simulink model "Drone_BBall_Developer"  (R2020a)
settings: Solver=FixedStepAuto  StartTime=0.0  StopTime=60  FixedStep=.001  RelTol=1e-3
values from neighbouring files (symbols this model uses):
  b = .25*m    (= 0.25)    [Run_Match.m]
  b_ball = .02*m_ball    (= 0.01)    [Run_Match.m]
  b_F_hook = 100    [Run_Match.m]
  b_F_hoop = m_ball * 50    (= 25)    [Run_Match.m]
  b_F_R = m * 20    (= 20)    [Run_Match.m]
  b_F_R_ball = m_ball * 10    (= 5)    [Run_Match.m]
  b_F_R_hook = m_hook * 100    (= 10)    [Run_Match.m]
  B_hook = r_hook^2*6*m_ball*g    (= 0.2943)    [Run_Match.m]
  b_hook = 0.05*m_hook    (= 0.005)    [Run_Match.m]
  b_tether = 1    [Run_Match.m]
  b_th = .1*J    (= 0.0192708333333)    [Run_Match.m]
  b_th_ball = .05*J_ball    (= 0.0009)    [Run_Match.m]
  b_x_net = 80*m_ball*g    (= 392.4)    [Run_Match.m]
  b_y_net = .4*m_ball*g    (= 1.962)    [Run_Match.m]
  drone = struct([])    [Run_Match.m]    (also in animate_drone_bball.m = [-r+w -r-w -r -r r r r+w r-w;             h    h  h  0 0 h  )
  g = 9.81    [Run_Match.m]
  J = 1/4*m*r^2 + 1/12*m*(2*(r+r_M_R))^2    (= 0.192708333333)    [Run_Match.m]
  J_ball = 2/5*m_ball*r_ball^2    (= 0.018)    [Run_Match.m]
  k_f = 4    [Run_Match.m]
  k_F_hook = 10000    [Run_Match.m]
  k_F_hoop = m_ball * 5000    (= 2500)    [Run_Match.m]
  k_F_R = m * 10000    (= 10000)    [Run_Match.m]
  k_F_R_ball = m_ball * 10000    (= 5000)    [Run_Match.m]
  k_F_R_hook = m_hook * 10000    (= 1000)    [Run_Match.m]
  k_tether = 40    [Run_Match.m]
  k_x_net = 200*m_ball*g    (= 981)    [Run_Match.m]
  k_y_net = .5*m_ball*g    (= 2.4525)    [Run_Match.m]
  L_tether = 1.0    (= 1)    [Run_Match.m]
  m = 1    [Run_Match.m]
  m_ball = .5    (= 0.5)    [Run_Match.m]
  m_hook = 0.1*m    (= 0.1)    [Run_Match.m]
  mu_f = .2    (= 0.2)    [Run_Match.m]
  mu_f_gnd = 0.5    [Run_Match.m]
  p_0 = [-5; 5]    [Run_Match.m]
  p_ball_0 = [0; r_ball]    [Run_Match.m]
  p_ball_dot_0 = [0; 12]    [Run_Match.m]
  p_emp = [0; -.4]    [Run_Match.m]
  p_emp_dot = [0; -5]    [Run_Match.m]
  p_hoop = [7.5 8; 8.5 8; -8.5 8; -7.5 8]'    [Run_Match.m]
  p_tether = [0; -0.259]    [Run_Match.m]
  r = 0.5    [Run_Match.m]    (also in animate_drone_bball.m = 0.475)
  r_ball = .3    (= 0.3)    [Run_Match.m]
  r_hook = 0.1    [Run_Match.m]
  r_M_R = 0.25*r    (= 0.125)    [Run_Match.m]
  T_0 = m*g    (= 9.81)    [Run_Match.m]
  T_max = 4*m*g    (= 39.24)    [Run_Match.m]
  T_tau = 0.1    [Run_Match.m]
undefined symbols (not defined in the file or in its folder): clock, M_max, sigbuilder_block, T_aux
libraries: dspswit3 x22, simulink x17, simulink_extras x3, dspmathops x2
(part 3 of 5)

== system Drone_BBall_Developer/EMP Mechanics//Dynamics/EMP Dynamics 1 ==
  Reset : Inport
  X_drone : Inport  Port=2
  Atan2 : Trigonometry  Operator=atan2
  Constant : Constant  Value=[0;0]
  Constant1 : Constant  Value=p_emp
  Constant2 : Constant  Value=p_emp_dot
  Constant3 : Constant  Value=0
  Demux : Demux  Outputs=2
  Demux1 : Demux  Outputs=6
  Demux2 : Demux  Outputs=2
  Demux3 : Demux  Outputs=2
  Gain : Gain  Gain=-1
  Integrator : Integrator  ExternalReset=level hold  InitialConditionSource=external  InitialCondition=p_ball_dot_0
  Integrator1 : Integrator  ExternalReset=level hold  InitialConditionSource=external  InitialCondition=p_ball_0
  Mux : Mux  Inputs=2
  Mux1 : Mux  Inputs=2
  Mux2 : Mux  Inputs=6
  Rotation Matrx : Subsystem
  Rotation Matrx1 : Subsystem
  Sum : Sum  Inputs=|++
  Sum1 : Sum  Inputs=|++
  Terminator : Terminator
  "X_emp " : Outport  VectorParamsAs1DForOutWhenUnconnected=off
  wires:
  Constant/1 -> Integrator/1
  Reset/1 -> Integrator1/2, Integrator/2
  Integrator/1 -> Demux/1, Demux3/1, Integrator1/1
  Integrator1/1 -> Demux2/1
  Atan2/1 -> Gain/1
  Demux/1 -> Atan2/2
  Demux/2 -> Atan2/1
  Constant1/1 -> Rotation Matrx/1(p)
  X_drone/1 -> Demux1/1
  Demux1/1 -> Mux/1
  Demux1/3 -> Mux/2
  Demux1/2 -> Mux1/1
  Demux1/4 -> Mux1/2
  Mux/1 -> Sum/1
  Demux1/5 -> Rotation Matrx1/2(theta), Rotation Matrx/2(theta)
  Rotation Matrx/1(R(theta)*p) -> Sum/2
  Sum/1 -> Integrator1/3
  Constant2/1 -> Rotation Matrx1/1(p)
  Mux1/1 -> Sum1/1
  Rotation Matrx1/1(R(theta)*p) -> Sum1/2
  Sum1/1 -> Integrator/3
  Demux1/6 -> Terminator/1
  Demux2/1 -> Mux2/1
  Demux3/1 -> Mux2/2
  Demux3/2 -> Mux2/4
  Demux2/2 -> Mux2/3
  Constant3/1 -> Mux2/6
  Mux2/1 -> "X_emp "/1
  Gain/1 -> Mux2/5

== system Drone_BBall_Developer/EMP Mechanics//Dynamics/EMP Dynamics 2 ==
  Reset : Inport
  X_drone : Inport  Port=2
  Atan2 : Trigonometry  Operator=atan2
  Constant : Constant  Value=[0;0]
  Constant1 : Constant  Value=p_emp
  Constant2 : Constant  Value=p_emp_dot
  Constant3 : Constant  Value=0
  Demux : Demux  Outputs=2
  Demux1 : Demux  Outputs=6
  Demux2 : Demux  Outputs=2
  Demux3 : Demux  Outputs=2
  Gain : Gain  Gain=-1
  Integrator : Integrator  ExternalReset=level hold  InitialConditionSource=external  InitialCondition=p_ball_dot_0
  Integrator1 : Integrator  ExternalReset=level hold  InitialConditionSource=external  InitialCondition=p_ball_0
  Mux : Mux  Inputs=2
  Mux1 : Mux  Inputs=2
  Mux2 : Mux  Inputs=6
  Rotation Matrx : Subsystem
  Rotation Matrx1 : Subsystem
  Sum : Sum  Inputs=|++
  Sum1 : Sum  Inputs=|++
  Terminator : Terminator
  "X_emp " : Outport  VectorParamsAs1DForOutWhenUnconnected=off
  wires:
  Constant/1 -> Integrator/1
  Reset/1 -> Integrator1/2, Integrator/2
  Integrator/1 -> Demux/1, Demux3/1, Integrator1/1
  Integrator1/1 -> Demux2/1
  Atan2/1 -> Gain/1
  Demux/1 -> Atan2/2
  Demux/2 -> Atan2/1
  Constant1/1 -> Rotation Matrx/1(p)
  X_drone/1 -> Demux1/1
  Demux1/1 -> Mux/1
  Demux1/3 -> Mux/2
  Demux1/2 -> Mux1/1
  Demux1/4 -> Mux1/2
  Mux/1 -> Sum/1
  Demux1/5 -> Rotation Matrx1/2(theta), Rotation Matrx/2(theta)
  Rotation Matrx/1(R(theta)*p) -> Sum/2
  Sum/1 -> Integrator1/3
  Constant2/1 -> Rotation Matrx1/1(p)
  Mux1/1 -> Sum1/1
  Rotation Matrx1/1(R(theta)*p) -> Sum1/2
  Sum1/1 -> Integrator/3
  Demux1/6 -> Terminator/1
  Demux2/1 -> Mux2/1
  Demux3/1 -> Mux2/2
  Demux3/2 -> Mux2/4
  Demux2/2 -> Mux2/3
  Constant3/1 -> Mux2/6
  Mux2/1 -> "X_emp "/1
  Gain/1 -> Mux2/5

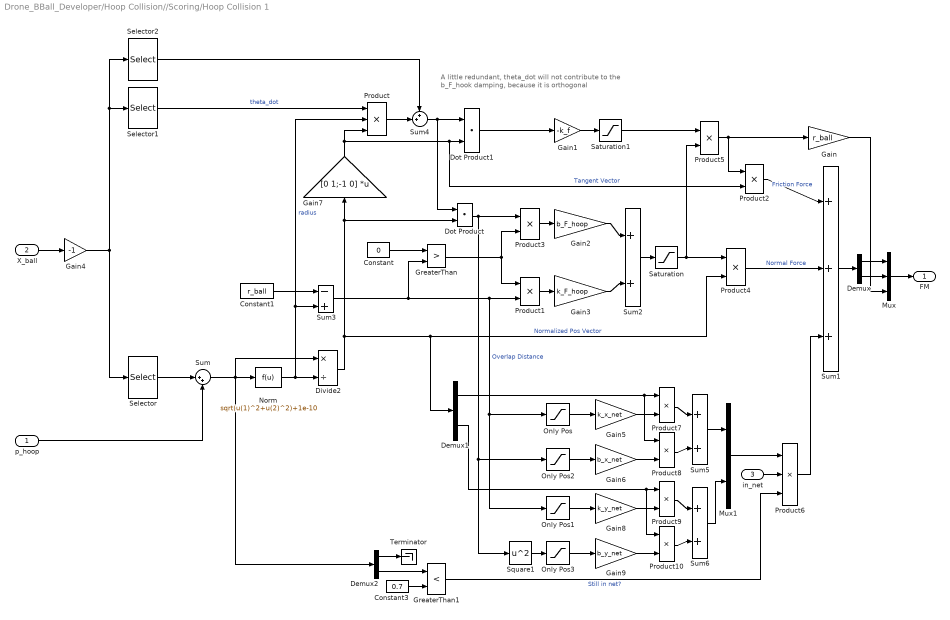
== system Drone_BBall_Developer/Hoop Collision//Scoring/Hoop Collision 1 ==
  note: A little redundant, theta_dot will not contribute to the
      | b_F_hook damping, because it is orthogonal
  p_hoop : Inport
  X_ball : Inport  Port=2
  in_net : Inport  Port=3
  Constant : Constant  Value=0
  Constant1 : Constant  Value=r_ball
  Constant3 : Constant  Value=0.7
  Demux : Demux  Outputs=2
  Demux1 : Demux  Outputs=2
  Demux2 : Demux  Outputs=2
  Divide2 : Product  Inputs=*/
  Dot Product : DotProduct  InputSameDT=on  OutDataTypeStr=Inherit: Inherit via internal rule
  Dot Product1 : DotProduct  InputSameDT=on  OutDataTypeStr=Inherit: Inherit via internal rule
  Gain : Gain  Gain=r_ball
  Gain1 : Gain  Gain=-k_f
  Gain2 : Gain  Gain=b_F_hoop
  Gain3 : Gain  Gain=k_F_hoop
  Gain4 : Gain  Gain=-1
  Gain5 : Gain  Gain=k_x_net
  Gain6 : Gain  Gain=b_x_net
  Gain7 : Gain  Gain=[0 1;-1 0]  Multiplication=Matrix(K*u)
  Gain8 : Gain  Gain=k_y_net
  Gain9 : Gain  Gain=b_y_net
  GreaterThan : RelationalOperator  Operator=>  OutDataTypeStr=boolean  RndMeth=Simplest
  GreaterThan1 : RelationalOperator  Operator=<  OutDataTypeStr=boolean  RndMeth=Simplest
  Mux : Mux  Inputs=3
  Mux1 : Mux  Inputs=2
  Norm : Fcn  Expr=sqrt(u(1)^2+u(2)^2)+1e-10
  Only Pos{,1..3} (4 alike) : Saturate  UpperLimit=Inf  LowerLimit=0
  Product : Product  Inputs=3
  Product{1..5,7..10} (9 alike) : Product
  Product6 : Product  Inputs=3
  Saturation : Saturate  UpperLimit=0  LowerLimit=-Inf
  Saturation1 : Saturate  UpperLimit=mu_f  LowerLimit=-mu_f
  Selector : Selector  InputPortWidth=6  IndexOptions=Index vector (dialog)  Indices=[1 3]  OutputSizes=1
  Selector1 : Selector  InputPortWidth=6  IndexOptions=Index vector (dialog)  Indices=[6]  OutputSizes=1
  Selector2 : Selector  InputPortWidth=6  IndexOptions=Index vector (dialog)  Indices=[2 4]  OutputSizes=1
  Square1 : Math  Operator=square  SignedPower=on  SaturateOnIntegerOverflow=on
  Sum : Sum  Inputs=|++
  Sum1 : Sum  Inputs=+||+||+
  Sum2 : Sum  Inputs=+|+
  Sum3 : Sum  Inputs=-|+
  Sum4 : Sum  Inputs=++|
  Sum5 : Sum  Inputs=+|+
  Sum6 : Sum  Inputs=+|+
  Terminator : Terminator
  FM : Outport  VectorParamsAs1DForOutWhenUnconnected=off
  wires:
  Gain/1 -> Mux/3
  p_hoop/1 -> Sum/2
  X_ball/1 -> Gain4/1
  Gain4/1 -> Selector1/1, Selector2/1, Selector/1
  Sum/1 -> Demux2/1, Divide2/1, Norm/1
  Sum3/1 -> Product1/2, Only Pos/1, Only Pos1/1, GreaterThan/2  "Overlap Distance"
  Constant/1 -> GreaterThan/1
  GreaterThan/1 -> Product1/1, Product3/2
  Product3/1 -> Gain2/1
  Dot Product1/1 -> Gain1/1
  Gain2/1 -> Sum2/1
  Gain3/1 -> Sum2/2
  Product5/1 -> Product2/1, Gain/1
  Norm/1 -> Product/2, Sum3/2, Divide2/2  "radius"
  Constant1/1 -> Sum3/1
  Divide2/1 -> Demux1/1, Product4/2, Gain7/1, Dot Product/2  "Normalized Pos Vector"
  Product1/1 -> Gain3/1
  Gain7/1 -> Product/3, Product2/2, Dot Product1/2  "Tangent Vector"
  Product/1 -> Sum4/2
  Selector2/1 -> Sum4/1
  Sum4/1 -> Dot Product/1, Dot Product1/1
  Selector1/1 -> Product/1  "theta_dot"
  Gain1/1 -> Saturation1/1
  Product4/1 -> Sum1/2  "Normal Force"
  Product2/1 -> Sum1/1  "Friction Force"
  Saturation/1 -> Product5/2, Product4/1
  Sum2/1 -> Saturation/1
  Saturation1/1 -> Product5/1
  Selector/1 -> Sum/1
  Mux/1 -> FM/1
  Sum1/1 -> Demux/1
  Demux/1 -> Mux/1
  Demux/2 -> Mux/2
  Only Pos/1 -> Gain5/1
  Only Pos2/1 -> Gain6/1
  Constant3/1 -> GreaterThan1/2
  Demux2/1 -> Terminator/1
  Demux2/2 -> GreaterThan1/1
  GreaterThan1/1 -> Product6/3  "Still in net?"
  Product6/1 -> Sum1/3
  Gain5/1 -> Product7/2
  Gain6/1 -> Product8/2
  Product7/1 -> Sum5/1
  Product8/1 -> Sum5/2
  Dot Product/1 -> Only Pos2/1, Square1/1, Product3/1
  Demux1/1 -> Product8/1, Product7/1
  Gain9/1 -> Product10/2
  Only Pos3/1 -> Gain9/1
  Product10/1 -> Sum6/2
  Square1/1 -> Only Pos3/1
  Demux1/2 -> Product10/1, Product9/1
  Gain8/1 -> Product9/2
  Only Pos1/1 -> Gain8/1
  Product9/1 -> Sum6/1
  Sum5/1 -> Mux1/1
  Sum6/1 -> Mux1/2
  Mux1/1 -> Product6/1
  in_net/1 -> Product6/2

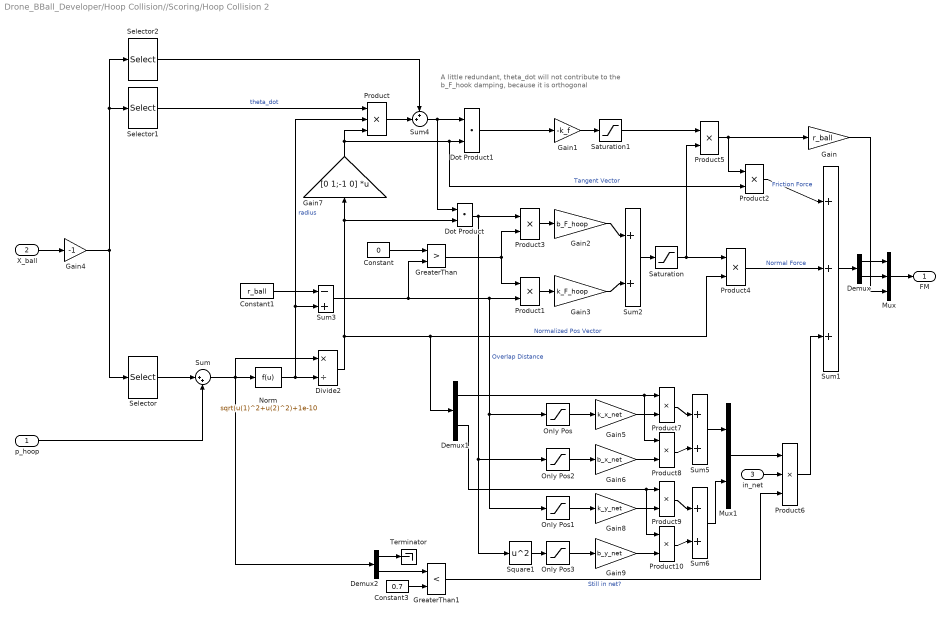
== system Drone_BBall_Developer/Hoop Collision//Scoring/Hoop Collision 2 ==
  note: A little redundant, theta_dot will not contribute to the
      | b_F_hook damping, because it is orthogonal
  p_hoop : Inport
  X_ball : Inport  Port=2
  in_net : Inport  Port=3
  Constant : Constant  Value=0
  Constant1 : Constant  Value=r_ball
  Constant3 : Constant  Value=0.7
  Demux : Demux  Outputs=2
  Demux1 : Demux  Outputs=2
  Demux2 : Demux  Outputs=2
  Divide2 : Product  Inputs=*/
  Dot Product : DotProduct  InputSameDT=on  OutDataTypeStr=Inherit: Inherit via internal rule
  Dot Product1 : DotProduct  InputSameDT=on  OutDataTypeStr=Inherit: Inherit via internal rule
  Gain : Gain  Gain=r_ball
  Gain1 : Gain  Gain=-k_f
  Gain2 : Gain  Gain=b_F_hoop
  Gain3 : Gain  Gain=k_F_hoop
  Gain4 : Gain  Gain=-1
  Gain5 : Gain  Gain=k_x_net
  Gain6 : Gain  Gain=b_x_net
  Gain7 : Gain  Gain=[0 1;-1 0]  Multiplication=Matrix(K*u)
  Gain8 : Gain  Gain=k_y_net
  Gain9 : Gain  Gain=b_y_net
  GreaterThan : RelationalOperator  Operator=>  OutDataTypeStr=boolean  RndMeth=Simplest
  GreaterThan1 : RelationalOperator  Operator=<  OutDataTypeStr=boolean  RndMeth=Simplest
  Mux : Mux  Inputs=3
  Mux1 : Mux  Inputs=2
  Norm : Fcn  Expr=sqrt(u(1)^2+u(2)^2)+1e-10
  Only Pos{,1..3} (4 alike) : Saturate  UpperLimit=Inf  LowerLimit=0
  Product : Product  Inputs=3
  Product{1..5,7..10} (9 alike) : Product
  Product6 : Product  Inputs=3
  Saturation : Saturate  UpperLimit=0  LowerLimit=-Inf
  Saturation1 : Saturate  UpperLimit=mu_f  LowerLimit=-mu_f
  Selector : Selector  InputPortWidth=6  IndexOptions=Index vector (dialog)  Indices=[1 3]  OutputSizes=1
  Selector1 : Selector  InputPortWidth=6  IndexOptions=Index vector (dialog)  Indices=[6]  OutputSizes=1
  Selector2 : Selector  InputPortWidth=6  IndexOptions=Index vector (dialog)  Indices=[2 4]  OutputSizes=1
  Square1 : Math  Operator=square  SignedPower=on  SaturateOnIntegerOverflow=on
  Sum : Sum  Inputs=|++
  Sum1 : Sum  Inputs=+||+||+
  Sum2 : Sum  Inputs=+|+
  Sum3 : Sum  Inputs=-|+
  Sum4 : Sum  Inputs=++|
  Sum5 : Sum  Inputs=+|+
  Sum6 : Sum  Inputs=+|+
  Terminator : Terminator
  FM : Outport  VectorParamsAs1DForOutWhenUnconnected=off
  wires:
  Gain/1 -> Mux/3
  p_hoop/1 -> Sum/2
  X_ball/1 -> Gain4/1
  Gain4/1 -> Selector1/1, Selector2/1, Selector/1
  Sum/1 -> Demux2/1, Divide2/1, Norm/1
  Sum3/1 -> Product1/2, Only Pos/1, Only Pos1/1, GreaterThan/2  "Overlap Distance"
  Constant/1 -> GreaterThan/1
  GreaterThan/1 -> Product1/1, Product3/2
  Product3/1 -> Gain2/1
  Dot Product1/1 -> Gain1/1
  Gain2/1 -> Sum2/1
  Gain3/1 -> Sum2/2
  Product5/1 -> Product2/1, Gain/1
  Norm/1 -> Product/2, Sum3/2, Divide2/2  "radius"
  Constant1/1 -> Sum3/1
  Divide2/1 -> Demux1/1, Product4/2, Gain7/1, Dot Product/2  "Normalized Pos Vector"
  Product1/1 -> Gain3/1
  Gain7/1 -> Product/3, Product2/2, Dot Product1/2  "Tangent Vector"
  Product/1 -> Sum4/2
  Selector2/1 -> Sum4/1
  Sum4/1 -> Dot Product/1, Dot Product1/1
  Selector1/1 -> Product/1  "theta_dot"
  Gain1/1 -> Saturation1/1
  Product4/1 -> Sum1/2  "Normal Force"
  Product2/1 -> Sum1/1  "Friction Force"
  Saturation/1 -> Product5/2, Product4/1
  Sum2/1 -> Saturation/1
  Saturation1/1 -> Product5/1
  Selector/1 -> Sum/1
  Mux/1 -> FM/1
  Sum1/1 -> Demux/1
  Demux/1 -> Mux/1
  Demux/2 -> Mux/2
  Only Pos/1 -> Gain5/1
  Only Pos2/1 -> Gain6/1
  Constant3/1 -> GreaterThan1/2
  Demux2/1 -> Terminator/1
  Demux2/2 -> GreaterThan1/1
  GreaterThan1/1 -> Product6/3  "Still in net?"
  Product6/1 -> Sum1/3
  Gain5/1 -> Product7/2
  Gain6/1 -> Product8/2
  Product7/1 -> Sum5/1
  Product8/1 -> Sum5/2
  Dot Product/1 -> Only Pos2/1, Square1/1, Product3/1
  Demux1/1 -> Product8/1, Product7/1
  Gain9/1 -> Product10/2
  Only Pos3/1 -> Gain9/1
  Product10/1 -> Sum6/2
  Square1/1 -> Only Pos3/1
  Demux1/2 -> Product10/1, Product9/1
  Gain8/1 -> Product9/2
  Only Pos1/1 -> Gain8/1
  Product9/1 -> Sum6/1
  Sum5/1 -> Mux1/1
  Sum6/1 -> Mux1/2
  Mux1/1 -> Product6/1
  in_net/1 -> Product6/2

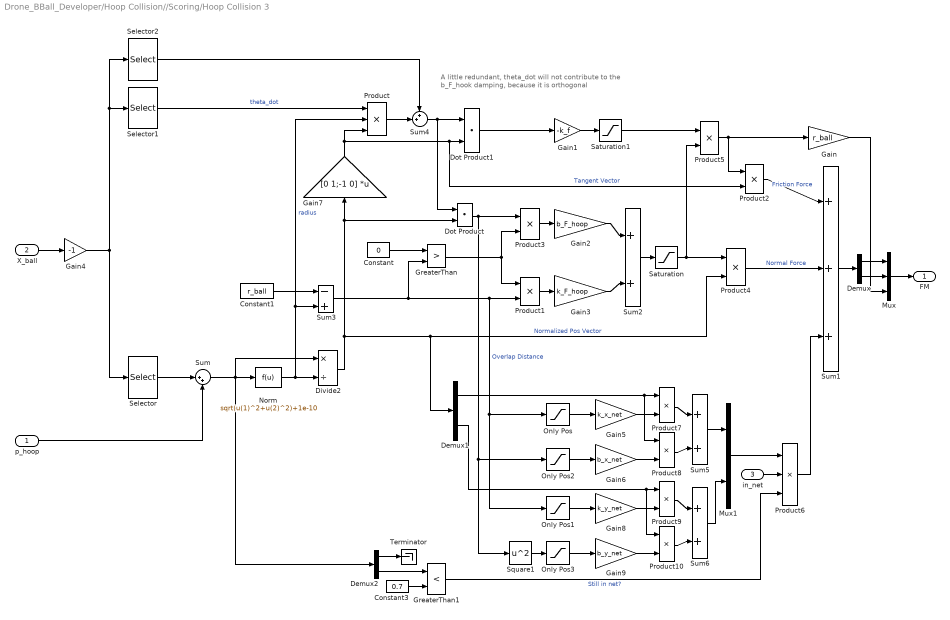
== system Drone_BBall_Developer/Hoop Collision//Scoring/Hoop Collision 3 ==
  note: A little redundant, theta_dot will not contribute to the
      | b_F_hook damping, because it is orthogonal
  p_hoop : Inport
  X_ball : Inport  Port=2
  in_net : Inport  Port=3
  Constant : Constant  Value=0
  Constant1 : Constant  Value=r_ball
  Constant3 : Constant  Value=0.7
  Demux : Demux  Outputs=2
  Demux1 : Demux  Outputs=2
  Demux2 : Demux  Outputs=2
  Divide2 : Product  Inputs=*/
  Dot Product : DotProduct  InputSameDT=on  OutDataTypeStr=Inherit: Inherit via internal rule
  Dot Product1 : DotProduct  InputSameDT=on  OutDataTypeStr=Inherit: Inherit via internal rule
  Gain : Gain  Gain=r_ball
  Gain1 : Gain  Gain=-k_f
  Gain2 : Gain  Gain=b_F_hoop
  Gain3 : Gain  Gain=k_F_hoop
  Gain4 : Gain  Gain=-1
  Gain5 : Gain  Gain=k_x_net
  Gain6 : Gain  Gain=b_x_net
  Gain7 : Gain  Gain=[0 1;-1 0]  Multiplication=Matrix(K*u)
  Gain8 : Gain  Gain=k_y_net
  Gain9 : Gain  Gain=b_y_net
  GreaterThan : RelationalOperator  Operator=>  OutDataTypeStr=boolean  RndMeth=Simplest
  GreaterThan1 : RelationalOperator  Operator=<  OutDataTypeStr=boolean  RndMeth=Simplest
  Mux : Mux  Inputs=3
  Mux1 : Mux  Inputs=2
  Norm : Fcn  Expr=sqrt(u(1)^2+u(2)^2)+1e-10
  Only Pos{,1..3} (4 alike) : Saturate  UpperLimit=Inf  LowerLimit=0
  Product : Product  Inputs=3
  Product{1..5,7..10} (9 alike) : Product
  Product6 : Product  Inputs=3
  Saturation : Saturate  UpperLimit=0  LowerLimit=-Inf
  Saturation1 : Saturate  UpperLimit=mu_f  LowerLimit=-mu_f
  Selector : Selector  InputPortWidth=6  IndexOptions=Index vector (dialog)  Indices=[1 3]  OutputSizes=1
  Selector1 : Selector  InputPortWidth=6  IndexOptions=Index vector (dialog)  Indices=[6]  OutputSizes=1
  Selector2 : Selector  InputPortWidth=6  IndexOptions=Index vector (dialog)  Indices=[2 4]  OutputSizes=1
  Square1 : Math  Operator=square  SignedPower=on  SaturateOnIntegerOverflow=on
  Sum : Sum  Inputs=|++
  Sum1 : Sum  Inputs=+||+||+
  Sum2 : Sum  Inputs=+|+
  Sum3 : Sum  Inputs=-|+
  Sum4 : Sum  Inputs=++|
  Sum5 : Sum  Inputs=+|+
  Sum6 : Sum  Inputs=+|+
  Terminator : Terminator
  FM : Outport  VectorParamsAs1DForOutWhenUnconnected=off
  wires:
  Gain/1 -> Mux/3
  p_hoop/1 -> Sum/2
  X_ball/1 -> Gain4/1
  Gain4/1 -> Selector1/1, Selector2/1, Selector/1
  Sum/1 -> Demux2/1, Divide2/1, Norm/1
  Sum3/1 -> Product1/2, Only Pos/1, Only Pos1/1, GreaterThan/2  "Overlap Distance"
  Constant/1 -> GreaterThan/1
  GreaterThan/1 -> Product1/1, Product3/2
  Product3/1 -> Gain2/1
  Dot Product1/1 -> Gain1/1
  Gain2/1 -> Sum2/1
  Gain3/1 -> Sum2/2
  Product5/1 -> Product2/1, Gain/1
  Norm/1 -> Product/2, Sum3/2, Divide2/2  "radius"
  Constant1/1 -> Sum3/1
  Divide2/1 -> Demux1/1, Product4/2, Gain7/1, Dot Product/2  "Normalized Pos Vector"
  Product1/1 -> Gain3/1
  Gain7/1 -> Product/3, Product2/2, Dot Product1/2  "Tangent Vector"
  Product/1 -> Sum4/2
  Selector2/1 -> Sum4/1
  Sum4/1 -> Dot Product/1, Dot Product1/1
  Selector1/1 -> Product/1  "theta_dot"
  Gain1/1 -> Saturation1/1
  Product4/1 -> Sum1/2  "Normal Force"
  Product2/1 -> Sum1/1  "Friction Force"
  Saturation/1 -> Product5/2, Product4/1
  Sum2/1 -> Saturation/1
  Saturation1/1 -> Product5/1
  Selector/1 -> Sum/1
  Mux/1 -> FM/1
  Sum1/1 -> Demux/1
  Demux/1 -> Mux/1
  Demux/2 -> Mux/2
  Only Pos/1 -> Gain5/1
  Only Pos2/1 -> Gain6/1
  Constant3/1 -> GreaterThan1/2
  Demux2/1 -> Terminator/1
  Demux2/2 -> GreaterThan1/1
  GreaterThan1/1 -> Product6/3  "Still in net?"
  Product6/1 -> Sum1/3
  Gain5/1 -> Product7/2
  Gain6/1 -> Product8/2
  Product7/1 -> Sum5/1
  Product8/1 -> Sum5/2
  Dot Product/1 -> Only Pos2/1, Square1/1, Product3/1
  Demux1/1 -> Product8/1, Product7/1
  Gain9/1 -> Product10/2
  Only Pos3/1 -> Gain9/1
  Product10/1 -> Sum6/2
  Square1/1 -> Only Pos3/1
  Demux1/2 -> Product10/1, Product9/1
  Gain8/1 -> Product9/2
  Only Pos1/1 -> Gain8/1
  Product9/1 -> Sum6/1
  Sum5/1 -> Mux1/1
  Sum6/1 -> Mux1/2
  Mux1/1 -> Product6/1
  in_net/1 -> Product6/2

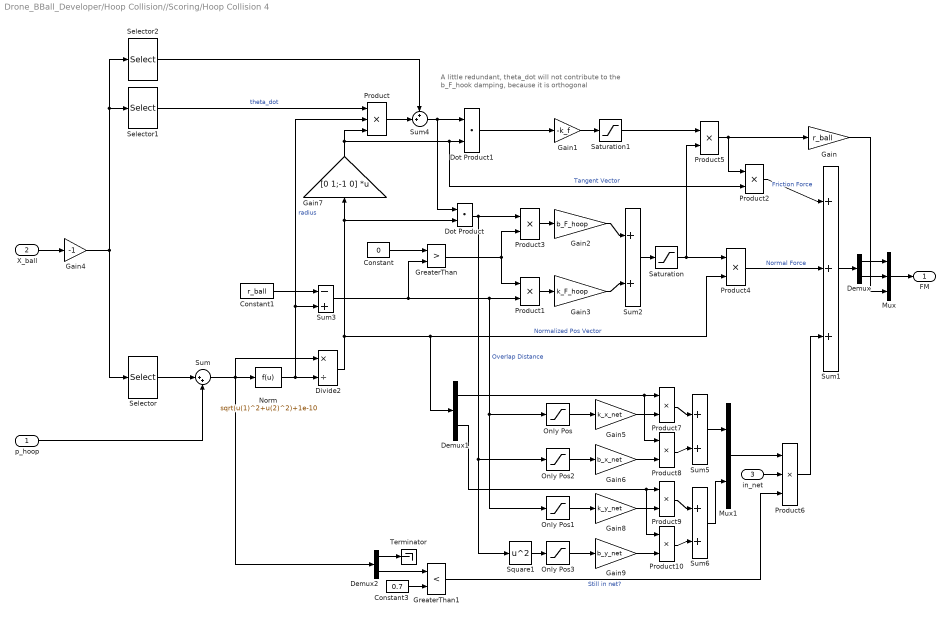
== system Drone_BBall_Developer/Hoop Collision//Scoring/Hoop Collision 4 ==
  note: A little redundant, theta_dot will not contribute to the
      | b_F_hook damping, because it is orthogonal
  p_hoop : Inport
  X_ball : Inport  Port=2
  in_net : Inport  Port=3
  Constant : Constant  Value=0
  Constant1 : Constant  Value=r_ball
  Constant3 : Constant  Value=0.7
  Demux : Demux  Outputs=2
  Demux1 : Demux  Outputs=2
  Demux2 : Demux  Outputs=2
  Divide2 : Product  Inputs=*/
  Dot Product : DotProduct  InputSameDT=on  OutDataTypeStr=Inherit: Inherit via internal rule
  Dot Product1 : DotProduct  InputSameDT=on  OutDataTypeStr=Inherit: Inherit via internal rule
  Gain : Gain  Gain=r_ball
  Gain1 : Gain  Gain=-k_f
  Gain2 : Gain  Gain=b_F_hoop
  Gain3 : Gain  Gain=k_F_hoop
  Gain4 : Gain  Gain=-1
  Gain5 : Gain  Gain=k_x_net
  Gain6 : Gain  Gain=b_x_net
  Gain7 : Gain  Gain=[0 1;-1 0]  Multiplication=Matrix(K*u)
  Gain8 : Gain  Gain=k_y_net
  Gain9 : Gain  Gain=b_y_net
  GreaterThan : RelationalOperator  Operator=>  OutDataTypeStr=boolean  RndMeth=Simplest
  GreaterThan1 : RelationalOperator  Operator=<  OutDataTypeStr=boolean  RndMeth=Simplest
  Mux : Mux  Inputs=3
  Mux1 : Mux  Inputs=2
  Norm : Fcn  Expr=sqrt(u(1)^2+u(2)^2)+1e-10
  Only Pos{,1..3} (4 alike) : Saturate  UpperLimit=Inf  LowerLimit=0
  Product : Product  Inputs=3
  Product{1..5,7..10} (9 alike) : Product
  Product6 : Product  Inputs=3
  Saturation : Saturate  UpperLimit=0  LowerLimit=-Inf
  Saturation1 : Saturate  UpperLimit=mu_f  LowerLimit=-mu_f
  Selector : Selector  InputPortWidth=6  IndexOptions=Index vector (dialog)  Indices=[1 3]  OutputSizes=1
  Selector1 : Selector  InputPortWidth=6  IndexOptions=Index vector (dialog)  Indices=[6]  OutputSizes=1
  Selector2 : Selector  InputPortWidth=6  IndexOptions=Index vector (dialog)  Indices=[2 4]  OutputSizes=1
  Square1 : Math  Operator=square  SignedPower=on  SaturateOnIntegerOverflow=on
  Sum : Sum  Inputs=|++
  Sum1 : Sum  Inputs=+||+||+
  Sum2 : Sum  Inputs=+|+
  Sum3 : Sum  Inputs=-|+
  Sum4 : Sum  Inputs=++|
  Sum5 : Sum  Inputs=+|+
  Sum6 : Sum  Inputs=+|+
  Terminator : Terminator
  FM : Outport  VectorParamsAs1DForOutWhenUnconnected=off
  wires:
  Gain/1 -> Mux/3
  p_hoop/1 -> Sum/2
  X_ball/1 -> Gain4/1
  Gain4/1 -> Selector1/1, Selector2/1, Selector/1
  Sum/1 -> Demux2/1, Divide2/1, Norm/1
  Sum3/1 -> Product1/2, Only Pos/1, Only Pos1/1, GreaterThan/2  "Overlap Distance"
  Constant/1 -> GreaterThan/1
  GreaterThan/1 -> Product1/1, Product3/2
  Product3/1 -> Gain2/1
  Dot Product1/1 -> Gain1/1
  Gain2/1 -> Sum2/1
  Gain3/1 -> Sum2/2
  Product5/1 -> Product2/1, Gain/1
  Norm/1 -> Product/2, Sum3/2, Divide2/2  "radius"
  Constant1/1 -> Sum3/1
  Divide2/1 -> Demux1/1, Product4/2, Gain7/1, Dot Product/2  "Normalized Pos Vector"
  Product1/1 -> Gain3/1
  Gain7/1 -> Product/3, Product2/2, Dot Product1/2  "Tangent Vector"
  Product/1 -> Sum4/2
  Selector2/1 -> Sum4/1
  Sum4/1 -> Dot Product/1, Dot Product1/1
  Selector1/1 -> Product/1  "theta_dot"
  Gain1/1 -> Saturation1/1
  Product4/1 -> Sum1/2  "Normal Force"
  Product2/1 -> Sum1/1  "Friction Force"
  Saturation/1 -> Product5/2, Product4/1
  Sum2/1 -> Saturation/1
  Saturation1/1 -> Product5/1
  Selector/1 -> Sum/1
  Mux/1 -> FM/1
  Sum1/1 -> Demux/1
  Demux/1 -> Mux/1
  Demux/2 -> Mux/2
  Only Pos/1 -> Gain5/1
  Only Pos2/1 -> Gain6/1
  Constant3/1 -> GreaterThan1/2
  Demux2/1 -> Terminator/1
  Demux2/2 -> GreaterThan1/1
  GreaterThan1/1 -> Product6/3  "Still in net?"
  Product6/1 -> Sum1/3
  Gain5/1 -> Product7/2
  Gain6/1 -> Product8/2
  Product7/1 -> Sum5/1
  Product8/1 -> Sum5/2
  Dot Product/1 -> Only Pos2/1, Square1/1, Product3/1
  Demux1/1 -> Product8/1, Product7/1
  Gain9/1 -> Product10/2
  Only Pos3/1 -> Gain9/1
  Product10/1 -> Sum6/2
  Square1/1 -> Only Pos3/1
  Demux1/2 -> Product10/1, Product9/1
  Gain8/1 -> Product9/2
  Only Pos1/1 -> Gain8/1
  Product9/1 -> Sum6/1
  Sum5/1 -> Mux1/1
  Sum6/1 -> Mux1/2
  Mux1/1 -> Product6/1
  in_net/1 -> Product6/2

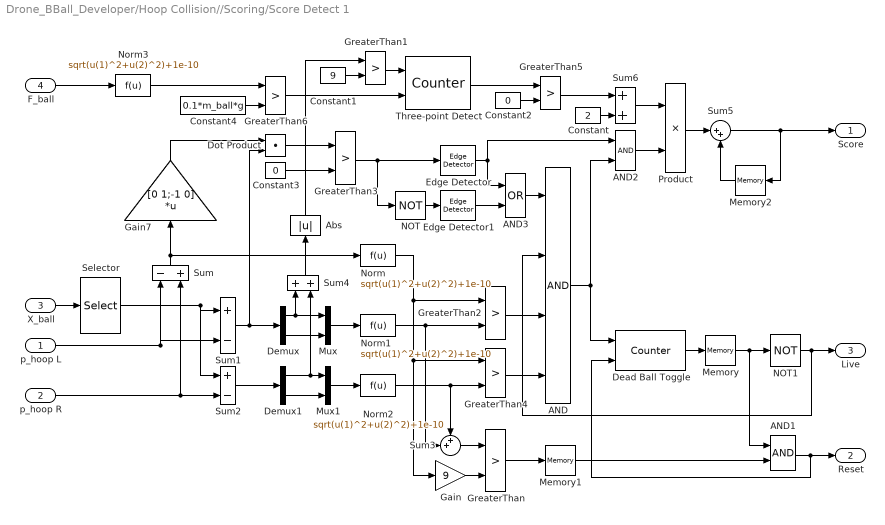
== system Drone_BBall_Developer/Hoop Collision//Scoring/Score Detect 1 ==
  p_hoop L : Inport
  p_hoop R : Inport  Port=2
  X_ball : Inport  Port=3
  F_ball : Inport  Port=4
  AND : Logic  Inputs=4  AllPortsSameDT=off  OutDataTypeStr=boolean
  AND1 : Logic  AllPortsSameDT=off  OutDataTypeStr=boolean
  AND2 : Logic  AllPortsSameDT=off  OutDataTypeStr=boolean
  AND3 : Logic  Operator=OR  AllPortsSameDT=off  OutDataTypeStr=boolean
  Abs : Abs
  Constant : Constant  Value=2
  Constant1 : Constant  Value=9
  Constant2 : Constant  Value=0
  Constant3 : Constant  Value=0
  Constant4 : Constant  Value=0.1*m_ball*g
  Dead Ball Toggle : dspswit3/Counter  Direction=Up  CountEvent=Rising edge  CounterSize=User defined  MaxCount=1  InitialCount=0  Output=Hit  HitValue=1  ResetInput=on  SamplesPerFrame=1  Ts=1  CntDtype=double  HitDtype=Logical
  Demux : Demux  Outputs=2
  Demux1 : Demux  Outputs=2
  Dot Product : DotProduct  InputSameDT=on  OutDataTypeStr=Inherit: Inherit via internal rule
  Edge Detector : dspswit3/Edge Detector
      settings: SourceProductBaseCode=DS
  Edge Detector1 : dspswit3/Edge Detector
      settings: SourceProductBaseCode=DS
  Gain : Gain  Gain=9
  Gain7 : Gain  Gain=[0 1;-1 0]  Multiplication=Matrix(K*u)
  GreaterThan{,1..6} (7 alike) : RelationalOperator  Operator=>  OutDataTypeStr=boolean  RndMeth=Simplest
  Memory : Memory
  Memory1 : Memory
  Memory2 : Memory
  Mux : Mux  Inputs=2
  Mux1 : Mux  Inputs=2
  NOT : Logic  Operator=NOT  IconShape=distinctive  AllPortsSameDT=off  OutDataTypeStr=boolean
  NOT1 : Logic  Operator=NOT  IconShape=distinctive  AllPortsSameDT=off  OutDataTypeStr=boolean
  Norm{,1..3} (4 alike) : Fcn  Expr=sqrt(u(1)^2+u(2)^2)+1e-10
  Product : Product
  Selector : Selector  InputPortWidth=6  IndexOptions=Index vector (dialog)  Indices=[1 3]  OutputSizes=1
  Sum : Sum  Inputs=-|+
  Sum1 : Sum  Inputs=+|-
  Sum2 : Sum  Inputs=+-
  Sum3 : Sum  Inputs=++|
  Sum4 : Sum
  Sum5 : Sum  Inputs=|++
  Sum6 : Sum  Inputs=+|+
  Three-point Detect : dspswit3/Counter  Direction=Up  CountEvent=Non-zero sample  CounterSize=User defined  MaxCount=1e10  InitialCount=0  Output=Count  HitValue=1  ResetInput=on  SamplesPerFrame=1  Ts=1  CntDtype=double  HitDtype=Logical
  Score : Outport  VectorParamsAs1DForOutWhenUnconnected=off
  Reset : Outport  Port=2  VectorParamsAs1DForOutWhenUnconnected=off
  Live : Outport  Port=3  VectorParamsAs1DForOutWhenUnconnected=off
  wires:
  Dot Product/1 -> GreaterThan3/1
  Sum/1 -> Norm/1, Gain7/1
  Norm1/1 -> GreaterThan2/2, Sum3/2
  Constant3/1 -> GreaterThan3/2
  Norm2/1 -> Sum3/1, GreaterThan4/2
  GreaterThan4/1 -> AND/4
  GreaterThan3/1 -> NOT/1, Edge Detector/1
  GreaterThan2/1 -> AND/3
  Gain7/1 -> Dot Product/1
  X_ball/1 -> Selector/1
  p_hoop L/1 -> Sum/1, Sum1/2
  p_hoop R/1 -> Sum/2, Sum2/2
  AND1/1 -> Reset/1, Dead Ball Toggle/2
  AND/1 -> AND2/2, Dead Ball Toggle/1
  Dead Ball Toggle/1 -> Memory/1
  Norm/1 -> GreaterThan2/1, GreaterThan4/1, Gain/1
  GreaterThan/1 -> Memory1/1
  Gain/1 -> GreaterThan/2
  Sum3/1 -> GreaterThan/1
  NOT1/1 -> AND/2, Live/1
  Memory/1 -> NOT1/1, AND1/1
  Memory1/1 -> AND1/2
  Demux/1 -> Mux/1, Sum4/1
  Demux/2 -> Mux/2
  Mux/1 -> Norm1/1
  Selector/1 -> Sum1/1, Sum2/1
  Demux1/2 -> Mux1/2
  Demux1/1 -> Sum4/2, Mux1/1
  Sum1/1 -> Demux/1, Dot Product/2
  Sum2/1 -> Demux1/1
  Mux1/1 -> Norm2/1
  Edge Detector/1 -> AND2/1, AND3/1
  NOT/1 -> Edge Detector1/1
  Edge Detector1/1 -> AND3/2
  AND3/1 -> AND/1
  Sum4/1 -> Abs/1
  Abs/1 -> GreaterThan1/1
  Constant1/1 -> GreaterThan1/2
  GreaterThan1/1 -> Three-point Detect/1
  F_ball/1 -> Norm3/1
  GreaterThan6/1 -> Three-point Detect/2
  Sum5/1 -> Score/1, Memory2/1
  Memory2/1 -> Sum5/2
  AND2/1 -> Product/2
  Constant/1 -> Sum6/2
  Sum6/1 -> Product/1
  Product/1 -> Sum5/1
  Three-point Detect/1 -> GreaterThan5/1
  GreaterThan5/1 -> Sum6/1
  Constant2/1 -> GreaterThan5/2
  Norm3/1 -> GreaterThan6/1
  Constant4/1 -> GreaterThan6/2

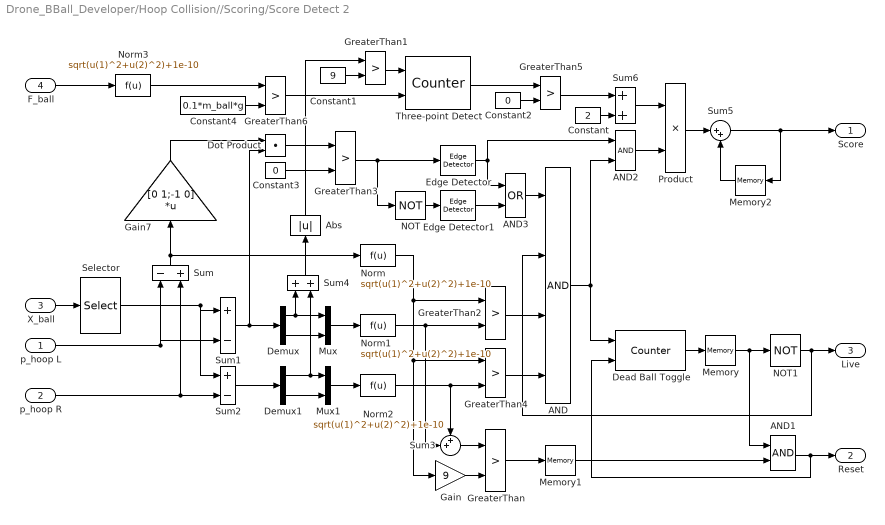
== system Drone_BBall_Developer/Hoop Collision//Scoring/Score Detect 2 ==
  p_hoop L : Inport
  p_hoop R : Inport  Port=2
  X_ball : Inport  Port=3
  F_ball : Inport  Port=4
  AND : Logic  Inputs=4  AllPortsSameDT=off  OutDataTypeStr=boolean
  AND1 : Logic  AllPortsSameDT=off  OutDataTypeStr=boolean
  AND2 : Logic  AllPortsSameDT=off  OutDataTypeStr=boolean
  AND3 : Logic  Operator=OR  AllPortsSameDT=off  OutDataTypeStr=boolean
  Abs : Abs
  Constant : Constant  Value=2
  Constant1 : Constant  Value=9
  Constant2 : Constant  Value=0
  Constant3 : Constant  Value=0
  Constant4 : Constant  Value=0.1*m_ball*g
  Dead Ball Toggle : dspswit3/Counter  Direction=Up  CountEvent=Rising edge  CounterSize=User defined  MaxCount=1  InitialCount=0  Output=Hit  HitValue=1  ResetInput=on  SamplesPerFrame=1  Ts=1  CntDtype=double  HitDtype=Logical
  Demux : Demux  Outputs=2
  Demux1 : Demux  Outputs=2
  Dot Product : DotProduct  InputSameDT=on  OutDataTypeStr=Inherit: Inherit via internal rule
  Edge Detector : dspswit3/Edge Detector
      settings: SourceProductBaseCode=DS
  Edge Detector1 : dspswit3/Edge Detector
      settings: SourceProductBaseCode=DS
  Gain : Gain  Gain=9
  Gain7 : Gain  Gain=[0 1;-1 0]  Multiplication=Matrix(K*u)
  GreaterThan{,1..6} (7 alike) : RelationalOperator  Operator=>  OutDataTypeStr=boolean  RndMeth=Simplest
  Memory : Memory
  Memory1 : Memory
  Memory2 : Memory
  Mux : Mux  Inputs=2
  Mux1 : Mux  Inputs=2
  NOT : Logic  Operator=NOT  IconShape=distinctive  AllPortsSameDT=off  OutDataTypeStr=boolean
  NOT1 : Logic  Operator=NOT  IconShape=distinctive  AllPortsSameDT=off  OutDataTypeStr=boolean
  Norm{,1..3} (4 alike) : Fcn  Expr=sqrt(u(1)^2+u(2)^2)+1e-10
  Product : Product
  Selector : Selector  InputPortWidth=6  IndexOptions=Index vector (dialog)  Indices=[1 3]  OutputSizes=1
  Sum : Sum  Inputs=-|+
  Sum1 : Sum  Inputs=+|-
  Sum2 : Sum  Inputs=+-
  Sum3 : Sum  Inputs=++|
  Sum4 : Sum
  Sum5 : Sum  Inputs=|++
  Sum6 : Sum  Inputs=+|+
  Three-point Detect : dspswit3/Counter  Direction=Up  CountEvent=Non-zero sample  CounterSize=User defined  MaxCount=1e10  InitialCount=0  Output=Count  HitValue=1  ResetInput=on  SamplesPerFrame=1  Ts=1  CntDtype=double  HitDtype=Logical
  Score : Outport  VectorParamsAs1DForOutWhenUnconnected=off
  Reset : Outport  Port=2  VectorParamsAs1DForOutWhenUnconnected=off
  Live : Outport  Port=3  VectorParamsAs1DForOutWhenUnconnected=off
  wires:
  Dot Product/1 -> GreaterThan3/1
  Sum/1 -> Norm/1, Gain7/1
  Norm1/1 -> GreaterThan2/2, Sum3/2
  Constant3/1 -> GreaterThan3/2
  Norm2/1 -> Sum3/1, GreaterThan4/2
  GreaterThan4/1 -> AND/4
  GreaterThan3/1 -> NOT/1, Edge Detector/1
  GreaterThan2/1 -> AND/3
  Gain7/1 -> Dot Product/1
  X_ball/1 -> Selector/1
  p_hoop L/1 -> Sum/1, Sum1/2
  p_hoop R/1 -> Sum/2, Sum2/2
  AND1/1 -> Reset/1, Dead Ball Toggle/2
  AND/1 -> AND2/2, Dead Ball Toggle/1
  Dead Ball Toggle/1 -> Memory/1
  Norm/1 -> GreaterThan2/1, GreaterThan4/1, Gain/1
  GreaterThan/1 -> Memory1/1
  Gain/1 -> GreaterThan/2
  Sum3/1 -> GreaterThan/1
  NOT1/1 -> AND/2, Live/1
  Memory/1 -> NOT1/1, AND1/1
  Memory1/1 -> AND1/2
  Demux/1 -> Mux/1, Sum4/1
  Demux/2 -> Mux/2
  Mux/1 -> Norm1/1
  Selector/1 -> Sum1/1, Sum2/1
  Demux1/2 -> Mux1/2
  Demux1/1 -> Sum4/2, Mux1/1
  Sum1/1 -> Demux/1, Dot Product/2
  Sum2/1 -> Demux1/1
  Mux1/1 -> Norm2/1
  Edge Detector/1 -> AND2/1, AND3/1
  NOT/1 -> Edge Detector1/1
  Edge Detector1/1 -> AND3/2
  AND3/1 -> AND/1
  Sum4/1 -> Abs/1
  Abs/1 -> GreaterThan1/1
  Constant1/1 -> GreaterThan1/2
  GreaterThan1/1 -> Three-point Detect/1
  F_ball/1 -> Norm3/1
  GreaterThan6/1 -> Three-point Detect/2
  Sum5/1 -> Score/1, Memory2/1
  Memory2/1 -> Sum5/2
  AND2/1 -> Product/2
  Constant/1 -> Sum6/2
  Sum6/1 -> Product/1
  Product/1 -> Sum5/1
  Three-point Detect/1 -> GreaterThan5/1
  GreaterThan5/1 -> Sum6/1
  Constant2/1 -> GreaterThan5/2
  Norm3/1 -> GreaterThan6/1
  Constant4/1 -> GreaterThan6/2

== system Drone_BBall_Developer/Qualification Drone Controller/__InputSSForSFun__ ==
  X_drone : Inport
  X_ball : Inport  Port=2
  X_opponent : Inport  Port=3
  F_tether : Inport  Port=4
  EMP armed : Inport  Port=5
  __UniqueOutportName__1__ : Outport
  __UniqueOutportName__2__ : Outport  Port=2
  __UniqueOutportName__3__ : Outport  Port=3
  __UniqueOutportName__4__ : Outport  Port=4
  __UniqueOutportName__5__ : Outport  Port=5
  wires:
  X_drone/1 -> __UniqueOutportName__1__/1
  X_ball/1 -> __UniqueOutportName__2__/1
  X_opponent/1 -> __UniqueOutportName__3__/1
  F_tether/1 -> __UniqueOutportName__4__/1
  EMP armed/1 -> __UniqueOutportName__5__/1

== system Drone_BBall_Developer/Qualification Drone Controller/__OutputSSForSFun__ ==
  __UniqueInportName__1__ : Inport
  __UniqueInportName__2__ : Inport  Port=2
  __UniqueInportName__3__ : Inport  Port=3
  __UniqueInportName__4__ : Inport  Port=4
  __UniqueInportName__5__ : Inport  Port=5
  fire_emp : Outport  VectorParamsAs1DForOutWhenUnconnected=off
  mag_on : Outport  Port=2  VectorParamsAs1DForOutWhenUnconnected=off
  T_L_d : Outport  Port=3  VectorParamsAs1DForOutWhenUnconnected=off
  T_R_d : Outport  Port=4  VectorParamsAs1DForOutWhenUnconnected=off
  X_d : Outport  Port=5  VectorParamsAs1DForOutWhenUnconnected=off
  wires:
  __UniqueInportName__1__/1 -> fire_emp/1
  __UniqueInportName__2__/1 -> mag_on/1
  __UniqueInportName__3__/1 -> T_L_d/1
  __UniqueInportName__4__/1 -> T_R_d/1
  __UniqueInportName__5__/1 -> X_d/1

== system Drone_BBall_Developer/Ball Dynamics/Rotational Dynamics/Wrap Angle ==
  raw : Inport
  Gain : Gain  Gain=2
  Mod : Math  Operator=mod  SignedPower=on  SaturateOnIntegerOverflow=on
  Pi : Constant  Value=pi  OutDataTypeStr=Inherit: Inherit via back propagation
  Sum3 : Sum  Inputs=|+-
  Sum4 : Sum  Inputs=|++
  wrap : Outport  VectorParamsAs1DForOutWhenUnconnected=off
  wires:
  Sum4/1 -> Mod/1
  Sum3/1 -> wrap/1
  raw/1 -> Sum4/1
  Mod/1 -> Sum3/1
  Gain/1 -> Mod/2
  Pi/1 -> Gain/1, Sum3/2, Sum4/2

== system Drone_BBall_Developer/Drone 1 Controller/Quadcopter Dynamical Controller/Diff btwn Angles ==
  theta : Inport
  theta_d : Inport  Port=2
  Sum5 : Sum  Inputs=-|+
  Wrap Angle : Subsystem
  e : Outport
  wires:
  theta/1 -> Sum5/1
  Sum5/1 -> Wrap Angle/1(raw)
  Wrap Angle/1(wrap) -> e/1
  theta_d/1 -> Sum5/2

== system Drone_BBall_Developer/Drone 1 Controller/Quadcopter Dynamical Controller/Thurst Mapping ==
  note: The first half of this subsystem
      | maps the desired net thrust and
      | net moment to the corresponding
      | desired left and right rotor thrust.
  note: The second half of this subsystem
      | creates a workaround for when the
      | desired thrust for either rotor is
      | negative (e.g., when trying to rotate
      | while the quadcopter is trying to fall).
      | The negative thrust in one rotor is
      | added as positive thrust to the other
      | rotor, allowing for rotation.
  note: The "Loop Break" linear analysis points are
      | necessary to linearize the y-axis dynamics
  M_d : Inport
  T_d : Inport  Port=2
  Gain : Gain  Gain=1/r
  Gain1 : Gain  Gain=1/2
  Gain2 : Gain  Gain=1/2
  Saturation : Saturate  UpperLimit=0  LowerLimit=-T_aux
  Saturation1 : Saturate  UpperLimit=0  LowerLimit=-T_aux
  Sum : Sum  Inputs=|++
  Sum1 : Sum  Inputs=+-|
  Sum2 : Sum  Inputs=|+-
  Sum3 : Sum  Inputs=-+|
  T_L_d : Outport  VectorParamsAs1DForOutWhenUnconnected=off
  T_R_d : Outport  Port=2  VectorParamsAs1DForOutWhenUnconnected=off
  wires:
  Gain/1 -> Sum/2, Sum1/2
  T_d/1 -> Sum1/1, Sum/1
  Sum/1 -> Gain1/1
  Sum1/1 -> Gain2/1
  M_d/1 -> Gain/1
  Gain1/1 -> Saturation/1, Sum2/1
  Sum2/1 -> T_L_d/1
  Sum3/1 -> T_R_d/1
  Gain2/1 -> Saturation1/1, Sum3/2
  Saturation/1 -> Sum3/1
  Saturation1/1 -> Sum2/2

== system Drone_BBall_Developer/Drone 1 Controller/Quadcopter Dynamical Controller/Wrap Angle ==
  raw : Inport
  Gain : Gain  Gain=2
  Mod : Math  Operator=mod  SignedPower=on  SaturateOnIntegerOverflow=on
  Pi : Constant  Value=pi  OutDataTypeStr=Inherit: Inherit via back propagation
  Sum3 : Sum  Inputs=|+-
  Sum4 : Sum  Inputs=|++
  wrap : Outport  VectorParamsAs1DForOutWhenUnconnected=off
  wires:
  Sum4/1 -> Mod/1
  Pi/1 -> Sum4/2, Sum3/2, Gain/1
  Sum3/1 -> wrap/1
  raw/1 -> Sum4/1
  Mod/1 -> Sum3/1
  Gain/1 -> Mod/2

== system Drone_BBall_Developer/Drone 1 Controller/Quadcopter Dynamical Controller (Arena Frame)/Diff btwn Angles ==
  theta : Inport
  theta_d : Inport  Port=2
  Sum5 : Sum  Inputs=-|+
  Wrap Angle : Subsystem
  e : Outport
  wires:
  theta/1 -> Sum5/1
  Sum5/1 -> Wrap Angle/1(raw)
  Wrap Angle/1(wrap) -> e/1
  theta_d/1 -> Sum5/2

== system Drone_BBall_Developer/Drone 1 Controller/Quadcopter Dynamical Controller (Arena Frame)/Thurst Mapping ==
  note: The first half of this subsystem
      | maps the desired net thrust and
      | net moment to the corresponding
      | desired left and right rotor thrust.
  note: The second half of this subsystem
      | creates a workaround for when the
      | desired thrust for either rotor is
      | negative (e.g., when trying to rotate
      | while the quadcopter is trying to fall).
      | The negative thrust in one rotor is
      | added as positive thrust to the other
      | rotor, allowing for rotation.
  note: The "Loop Break" linear analysis points are
      | necessary to linearize the y-axis dynamics
  M_d : Inport
  T_d : Inport  Port=2
  Gain : Gain  Gain=1/r
  Gain1 : Gain  Gain=1/2
  Gain2 : Gain  Gain=1/2
  Saturation : Saturate  UpperLimit=0  LowerLimit=-0.1
  Saturation1 : Saturate  UpperLimit=0  LowerLimit=-0.1
  Sum : Sum  Inputs=|++
  Sum1 : Sum  Inputs=+-|
  Sum2 : Sum  Inputs=|+-
  Sum3 : Sum  Inputs=-+|
  T_L_d : Outport  VectorParamsAs1DForOutWhenUnconnected=off
  T_R_d : Outport  Port=2  VectorParamsAs1DForOutWhenUnconnected=off
  wires:
  Gain/1 -> Sum/2, Sum1/2
  T_d/1 -> Sum1/1, Sum/1
  Sum/1 -> Gain1/1
  Sum1/1 -> Gain2/1
  M_d/1 -> Gain/1
  Gain1/1 -> Saturation/1, Sum2/1
  Sum2/1 -> T_L_d/1
  Sum3/1 -> T_R_d/1
  Gain2/1 -> Saturation1/1, Sum3/2
  Saturation/1 -> Sum3/1
  Saturation1/1 -> Sum2/2

== system Drone_BBall_Developer/Drone 1 Controller/Quadcopter Dynamical Controller (Arena Frame)/Wrap Angle ==
  raw : Inport
  Gain : Gain  Gain=2
  Mod : Math  Operator=mod  SignedPower=on  SaturateOnIntegerOverflow=on
  Pi : Constant  Value=pi  OutDataTypeStr=Inherit: Inherit via back propagation
  Sum3 : Sum  Inputs=|+-
  Sum4 : Sum  Inputs=|++
  wrap : Outport  VectorParamsAs1DForOutWhenUnconnected=off
  wires:
  Sum4/1 -> Mod/1
  Pi/1 -> Sum4/2, Sum3/2, Gain/1
  Sum3/1 -> wrap/1
  raw/1 -> Sum4/1
  Mod/1 -> Sum3/1
  Gain/1 -> Mod/2

== system Drone_BBall_Developer/Drone 1 Controller/Quadcopter Dynamical Controller (Drone Frame)/Diff btwn Angles ==
  theta : Inport
  theta_d : Inport  Port=2
  Sum5 : Sum  Inputs=-|+
  Wrap Angle : Subsystem
  e : Outport
  wires:
  theta/1 -> Sum5/1
  Sum5/1 -> Wrap Angle/1(raw)
  Wrap Angle/1(wrap) -> e/1
  theta_d/1 -> Sum5/2

== system Drone_BBall_Developer/Drone 1 Controller/Quadcopter Dynamical Controller (Drone Frame)/Rotate e (CCW) ==
  p : Inport
  theta : Inport  Port=2
  Cos : Trigonometry  Operator=cos
  Demux : Demux  Outputs=2
  Demux1 : Demux  Outputs=2
  Mux3 : Mux  Inputs=2
  Product : Product
  Product1 : Product
  Sin : Trigonometry
  Sum1 : Sum  Inputs=+-
  Sum2 : Sum
  R(theta)*p : Outport  VectorParamsAs1DForOutWhenUnconnected=off
  wires:
  p/1 -> Product/2, Product1/2
  Sum2/1 -> Mux3/2
  Sin/1 -> Product1/1
  theta/1 -> Cos/1, Sin/1
  Cos/1 -> Product/1
  Sum1/1 -> Mux3/1
  Mux3/1 -> R(theta)*p/1
  Product/1 -> Demux/1
  Product1/1 -> Demux1/1
  Demux/1 -> Sum1/1
  Demux1/2 -> Sum1/2
  Demux1/1 -> Sum2/2
  Demux/2 -> Sum2/1

== system Drone_BBall_Developer/Drone 1 Controller/Quadcopter Dynamical Controller (Drone Frame)/Rotate e_dot (CCW) ==
  p : Inport
  theta : Inport  Port=2
  Cos : Trigonometry  Operator=cos
  Demux : Demux  Outputs=2
  Demux1 : Demux  Outputs=2
  Mux3 : Mux  Inputs=2
  Product : Product
  Product1 : Product
  Sin : Trigonometry
  Sum1 : Sum  Inputs=+-
  Sum2 : Sum
  R(theta)*p : Outport  VectorParamsAs1DForOutWhenUnconnected=off
  wires:
  p/1 -> Product/2, Product1/2
  Sum2/1 -> Mux3/2
  Sin/1 -> Product1/1
  theta/1 -> Cos/1, Sin/1
  Cos/1 -> Product/1
  Sum1/1 -> Mux3/1
  Mux3/1 -> R(theta)*p/1
  Product/1 -> Demux/1
  Product1/1 -> Demux1/1
  Demux/1 -> Sum1/1
  Demux1/2 -> Sum1/2
  Demux1/1 -> Sum2/2
  Demux/2 -> Sum2/1

== system Drone_BBall_Developer/Drone 1 Controller/Quadcopter Dynamical Controller (Drone Frame)/Thurst Mapping ==
  note: The first half of this subsystem
      | maps the desired net thrust and
      | net moment to the corresponding
      | desired left and right rotor thrust.
  note: The second half of this subsystem
      | creates a workaround for when the
      | desired thrust for either rotor is
      | negative (e.g., when trying to rotate
      | while the quadcopter is trying to fall).
      | The negative thrust in one rotor is
      | added as positive thrust to the other
      | rotor, allowing for rotation.
  note: The "Loop Break" linear analysis points are
      | necessary to linearize the y-axis dynamics
  M_d : Inport
  T_d : Inport  Port=2
  Gain : Gain  Gain=1/r
  Gain1 : Gain  Gain=1/2
  Gain2 : Gain  Gain=1/2
  Saturation : Saturate  UpperLimit=0  LowerLimit=-0.1
  Saturation1 : Saturate  UpperLimit=0  LowerLimit=-0.1
  Sum : Sum  Inputs=|++
  Sum1 : Sum  Inputs=+-|
  Sum2 : Sum  Inputs=|+-
  Sum3 : Sum  Inputs=-+|
  T_L_d : Outport  VectorParamsAs1DForOutWhenUnconnected=off
  T_R_d : Outport  Port=2  VectorParamsAs1DForOutWhenUnconnected=off
  wires:
  Gain/1 -> Sum/2, Sum1/2
  T_d/1 -> Sum1/1, Sum/1
  Sum/1 -> Gain1/1
  Sum1/1 -> Gain2/1
  M_d/1 -> Gain/1
  Gain1/1 -> Saturation/1, Sum2/1
  Sum2/1 -> T_L_d/1
  Sum3/1 -> T_R_d/1
  Gain2/1 -> Saturation1/1, Sum3/2
  Saturation/1 -> Sum3/1
  Saturation1/1 -> Sum2/2

== system Drone_BBall_Developer/Drone 1 Controller/Quadcopter Dynamical Controller (Drone Frame)/Wrap Angle ==
  raw : Inport
  Gain : Gain  Gain=2
  Mod : Math  Operator=mod  SignedPower=on  SaturateOnIntegerOverflow=on
  Pi : Constant  Value=pi  OutDataTypeStr=Inherit: Inherit via back propagation
  Sum3 : Sum  Inputs=|+-
  Sum4 : Sum  Inputs=|++
  wrap : Outport  VectorParamsAs1DForOutWhenUnconnected=off
  wires:
  Sum4/1 -> Mod/1
  Pi/1 -> Sum4/2, Sum3/2, Gain/1
  Sum3/1 -> wrap/1
  raw/1 -> Sum4/1
  Mod/1 -> Sum3/1
  Gain/1 -> Mod/2

== system Drone_BBall_Developer/Drone 1 Controller/Quadcopter Dynamical Controller (Drone Frame)/X-Axis PID ==
  e : Inport
  e_dot : Inport  Port=2
  Deg2Rad : Gain  Gain=pi/180
  Derivative Gain : Gain  Gain=K_D
  Integral Gain : Gain  Gain=K_I
  Integrator : Integrator  UpperSaturationLimit=u_max  LowerSaturationLimit=-u_max
  Proportioanl Gain : Gain  Gain=K_P
  Saturation : Saturate  UpperLimit=u_max  LowerLimit=-u_max
  Scope : Scope  NumInputPorts=3
  Sum : Sum  Inputs=|+-
  Sum4 : Sum  Inputs=+|+|+
  Switch : Switch  Criteria=u2 ~= 0
  Zero1 : Constant  Value=0  OutDataTypeStr=Inherit: Inherit via back propagation
  u : Outport  VectorParamsAs1DForOutWhenUnconnected=off
  wires:
  Proportioanl Gain/1 -> Sum4/2, Scope/1
  e_dot/1 -> Derivative Gain/1
  Integrator/1 -> Sum4/1, Scope/2
  Sum4/1 -> Sum/2, Saturation/1
  e/1 -> Integral Gain/1, Proportioanl Gain/1
  Derivative Gain/1 -> Sum4/3, Scope/3
  Deg2Rad/1 -> u/1
  Saturation/1 -> Deg2Rad/1, Sum/1
  Switch/1 -> Integrator/1
  Integral Gain/1 -> Switch/3
  Sum/1 -> Switch/2
  Zero1/1 -> Switch/1

== system Drone_BBall_Developer/Drone 1 Controller/Quadcopter Dynamical Controller (Drone Frame)/Y-Axis PID ==
  e : Inport
  e_dot : Inport  Port=2
  Derivative Gain : Gain  Gain=K_D
  Integral Gain : Gain  Gain=K_I
  Integrator1 : Integrator  InitialCondition=u_0  UpperSaturationLimit=u_max  LowerSaturationLimit=-u_max
  Overall Gain : Gain
  Proportional Gain : Gain  Gain=K_P
  Saturation : Saturate  UpperLimit=u_max  LowerLimit=0
  Scope : Scope  NumInputPorts=3
  Sum : Sum  Inputs=|+-
  Sum1 : Sum  Inputs=+|+|+
  Switch : Switch  Criteria=u2 ~= 0
  Zero1 : Constant  Value=0  OutDataTypeStr=Inherit: Inherit via back propagation
  u : Outport  VectorParamsAs1DForOutWhenUnconnected=off
  wires:
  e_dot/1 -> Derivative Gain/1
  Sum1/1 -> Saturation/1, Sum/2
  e/1 -> Integral Gain/1, Proportional Gain/1
  Derivative Gain/1 -> Sum1/3, Scope/3
  Saturation/1 -> Sum/1, Overall Gain/1
  Integrator1/1 -> Sum1/1, Scope/2
  Proportional Gain/1 -> Scope/1, Sum1/2
  Sum/1 -> Switch/2
  Zero1/1 -> Switch/1
  Switch/1 -> Integrator1/1
  Integral Gain/1 -> Switch/3
  Overall Gain/1 -> u/1

== system Drone_BBall_Developer/Drone 1 Dynamics/Hook Plant/Ground Reactions ==
  X : Inport
  Constant1 : Constant  Value=0
  Demux : Demux  Outputs=6
  Gain : Gain  Gain=-k_F_R_hook
  Gain4 : Gain  Gain=-b_F_R_hook
  Gain6 : Gain  Gain=-k_f
  Less Than1 : RelationalOperator  Operator=>  OutDataTypeStr=boolean  RndMeth=Simplest
  Mux : Mux  Inputs=2
  Product2 : Product
  Product5 : Product  Inputs=3
  Saturation : Saturate  UpperLimit=Inf  LowerLimit=0
  Saturation1 : Saturate  UpperLimit=mu_f  LowerLimit=-mu_f
  Sum1 : Sum  Inputs=|++
  Terminator : Terminator
  Terminator1 : Terminator
  Terminator2 : Terminator
  F_R : Outport  VectorParamsAs1DForOutWhenUnconnected=off
  wires:
  Gain6/1 -> Saturation1/1
  Saturation1/1 -> Product5/1
  Saturation/1 -> Product2/2, Product5/2
  Demux/1 -> Terminator/1
  Mux/1 -> F_R/1
  Product2/1 -> Mux/2
  Demux/5 -> Terminator1/1
  Constant1/1 -> Less Than1/1
  Demux/3 -> Gain/1, Less Than1/2
  Product5/1 -> Mux/1
  Gain4/1 -> Sum1/2
  Less Than1/1 -> Product5/3, Product2/1
  Sum1/1 -> Saturation/1
  Demux/2 -> Gain6/1
  Demux/4 -> Gain4/1
  Gain/1 -> Sum1/1
  X/1 -> Demux/1
  Demux/6 -> Terminator2/1

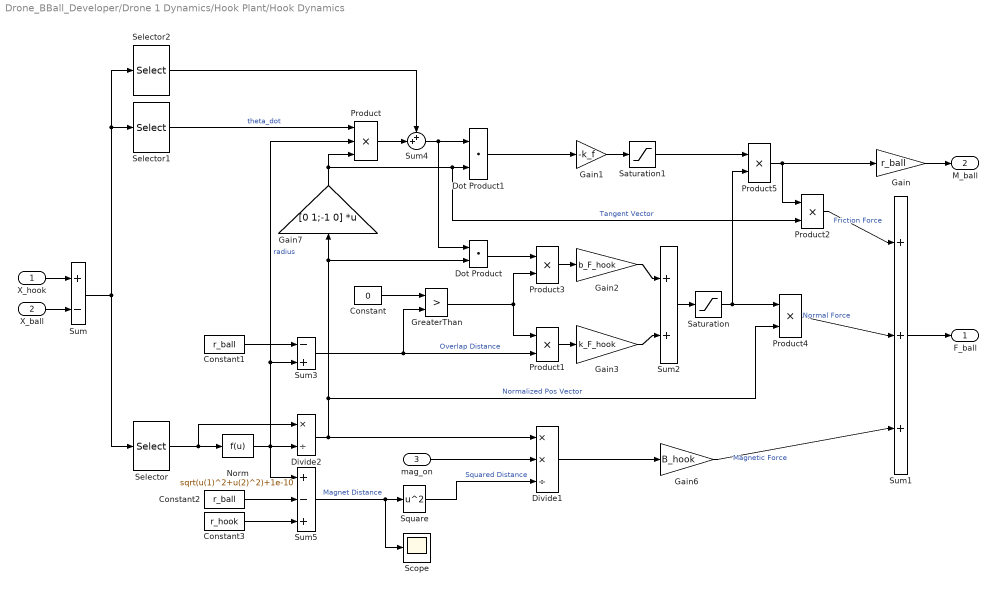
== system Drone_BBall_Developer/Drone 1 Dynamics/Hook Plant/Hook Dynamics ==
  X_hook : Inport
  X_ball : Inport  Port=2
  mag_on : Inport  Port=3
  Constant : Constant  Value=0
  Constant1 : Constant  Value=r_ball
  Constant2 : Constant  Value=r_ball
  Constant3 : Constant  Value=r_hook
  Divide1 : Product  Inputs=**/
  Divide2 : Product  Inputs=*/
  Dot Product : DotProduct  InputSameDT=on  OutDataTypeStr=Inherit: Inherit via internal rule
  Dot Product1 : DotProduct  InputSameDT=on  OutDataTypeStr=Inherit: Inherit via internal rule
  Gain : Gain  Gain=r_ball
  Gain1 : Gain  Gain=-k_f
  Gain2 : Gain  Gain=b_F_hook
  Gain3 : Gain  Gain=k_F_hook
  Gain6 : Gain  Gain=B_hook
  Gain7 : Gain  Gain=[0 1;-1 0]  Multiplication=Matrix(K*u)
  GreaterThan : RelationalOperator  Operator=>  OutDataTypeStr=boolean  RndMeth=Simplest
  Norm : Fcn  Expr=sqrt(u(1)^2+u(2)^2)+1e-10
  Product : Product  Inputs=3
  Product{1..5} (5 alike) : Product
  Saturation : Saturate  UpperLimit=0  LowerLimit=-Inf
  Saturation1 : Saturate  UpperLimit=mu_f  LowerLimit=-mu_f
  Scope : Scope
  Selector : Selector  InputPortWidth=6  IndexOptions=Index vector (dialog)  Indices=[1 3]  OutputSizes=1
  Selector1 : Selector  InputPortWidth=6  IndexOptions=Index vector (dialog)  Indices=[6]  OutputSizes=1
  Selector2 : Selector  InputPortWidth=6  IndexOptions=Index vector (dialog)  Indices=[2 4]  OutputSizes=1
  Square : Math  Operator=square  SignedPower=on  SaturateOnIntegerOverflow=on
  Sum : Sum  Inputs=+-
  Sum1 : Sum  Inputs=+||+|||+
  Sum2 : Sum  Inputs=+|+
  Sum3 : Sum  Inputs=-|+
  Sum4 : Sum  Inputs=++|
  Sum5 : Sum  Inputs=+-+
  F_ball : Outport  VectorParamsAs1DForOutWhenUnconnected=off
  M_ball : Outport  Port=2  VectorParamsAs1DForOutWhenUnconnected=off
  wires:
  Gain/1 -> M_ball/1
  mag_on/1 -> Divide1/2
  X_hook/1 -> Sum/1
  X_ball/1 -> Sum/2
  Sum/1 -> Selector1/1, Selector2/1, Selector/1
  Selector/1 -> Divide2/1, Norm/1
  Sum3/1 -> Product1/2, GreaterThan/2  "Overlap Distance"
  Constant/1 -> GreaterThan/1
  GreaterThan/1 -> Product1/1, Product3/2
  Product3/1 -> Gain2/1
  Sum1/1 -> F_ball/1
  Dot Product1/1 -> Gain1/1
  Gain2/1 -> Sum2/1
  Gain3/1 -> Sum2/2
  Product5/1 -> Product2/1, Gain/1
  Divide1/1 -> Gain6/1
  Gain6/1 -> Sum1/3  "Magnetic Force"
  Norm/1 -> Sum5/1, Divide2/2, Product/2, Sum3/2  "radius"
  Constant1/1 -> Sum3/1
  Divide2/1 -> Divide1/1, Product4/2, Gain7/1, Dot Product/2  "Normalized Pos Vector"
  Dot Product/1 -> Product3/1
  Product1/1 -> Gain3/1
  Square/1 -> Divide1/3  "Squared Distance"
  Gain7/1 -> Product/3, Product2/2, Dot Product1/2  "Tangent Vector"
  Product/1 -> Sum4/2
  Selector2/1 -> Sum4/1
  Sum4/1 -> Dot Product/1, Dot Product1/1
  Selector1/1 -> Product/1  "theta_dot"
  Gain1/1 -> Saturation1/1
  Product4/1 -> Sum1/2  "Normal Force"
  Product2/1 -> Sum1/1  "Friction Force"
  Saturation/1 -> Product5/2, Product4/1
  Sum2/1 -> Saturation/1
  Saturation1/1 -> Product5/1
  Constant2/1 -> Sum5/2
  Constant3/1 -> Sum5/3
  Sum5/1 -> Scope/1, Square/1  "Magnet Distance"

== system Drone_BBall_Developer/Drone 1 Dynamics/Hook Plant/Linear Dynamics ==
  F : Inport
  Gain : Gain  Gain=1/m_hook
  Gain1 : Gain  Gain=b_hook
  Integrator : Integrator  InitialCondition=param.X_0([1 3])+p_tether+[0;-L_tether]
  Integrator1 : Integrator  InitialCondition=param.X_0([2 4])
  Norm : Fcn  Expr=sqrt(u(1)^2+u(2)^2)
  Product : Product
  Sum3 : Sum  Inputs=+-
  p : Outport  VectorParamsAs1DForOutWhenUnconnected=off
  p_dot : Outport  Port=2  VectorParamsAs1DForOutWhenUnconnected=off
  wires:
  Gain1/1 -> Sum3/2
  Integrator1/1 -> Integrator/1, Norm/1, Product/1, p_dot/1
  Norm/1 -> Product/2
  Product/1 -> Gain1/1
  F/1 -> Sum3/1
  Sum3/1 -> Gain/1
  Gain/1 -> Integrator1/1
  Integrator/1 -> p/1
